simulink model "MinsegControlProjectSim"  (R2023a)
settings: Solver=FixedStepDiscrete  StartTime=0.0  StopTime=inf  FixedStep=0.03  RelTol=1e-3
values from neighbouring files (symbols this model uses):
  K_LQR = lqr(A,B,Q,R)    [MinsegControlProject.m]
libraries: arduinolib x2, RASPlib x2, simulink x1, MinSegLibrary_MinSegMega x1
settings Model: SimulationMode=external  ExtModeTrigDuration=2  Creator=nicho  LastModifiedBy=nicho
settings OptimizationCC: EnhancedBackFolding=on  PassReuseOutputArgsAs=Individual arguments  ZeroExternalMemoryAtStartup=off  ZeroInternalMemoryAtStartup=off  MaxStackSize=64  OptimizeBlockOrder=speed  DifferentSizesBufferReuse=on  OptimizationCustomize=off  EfficientTunableParamExpr=on
settings DebuggingCC: ParameterTunabilityLossMsg=error
settings HardwareCC: ProdBitPerInt=16  ProdBitPerPointer=16  ProdBitPerSizeT=16  ProdBitPerPtrDiffT=16  ProdLargestAtomicFloat=None  ProdWordSize=8  ProdHWDeviceType=Atmel->AVR  UseEmbeddedCoderFeatures=off  UseSimulinkCoderFeatures=off
settings SFSimCC: MATLABDynamicMemAlloc=off
settings RTWCC: Description=Embedded Coder  SystemTargetFile=ert.tlc  HardwareBoard=Arduino Mega 2560  TemplateMakefile=ert_default_tmf  RTWVerbose=off  Toolchain=Arduino AVR
settings CodeAppCC: ForceParamTrailComments=on  OperatorAnnotations=on  SimulinkDataObjDesc=on  SFDataObjDesc=on  MangleLength=10  InsertBlockDesc=on
settings ERTTargetCC: SupportContinuousTime=on  SupportNonInlinedSFcns=on  SupportVariableSizeSignals=on  ExtMode=on  ExtModeTransport=3  ExtModeStaticAlloc=on  ExtModeAutomaticAllocSize=off  ExtModeStaticAllocSize=2048  ExtModeMexFile=ext_xcp  ExtModeMexArgs=0 3 921600  ExtModeIntrfLevel=Level2 - Open  ERTSrcFileBannerTemplate=codertarget_code_template.cgt  ERTHdrFileBannerTemplate=codertarget_code_template.cgt  ERTDataSrcFileTemplate=codertarget_code_template.cgt  ERTDataHdrFileTemplate=codertarget_code_template.cgt

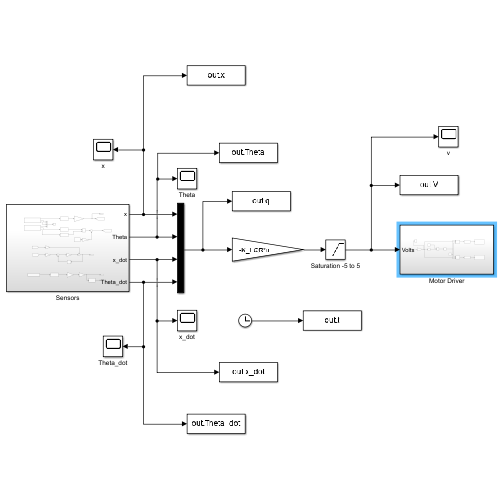
[thumbnail: Simulink's stored preview of the top-level diagram]
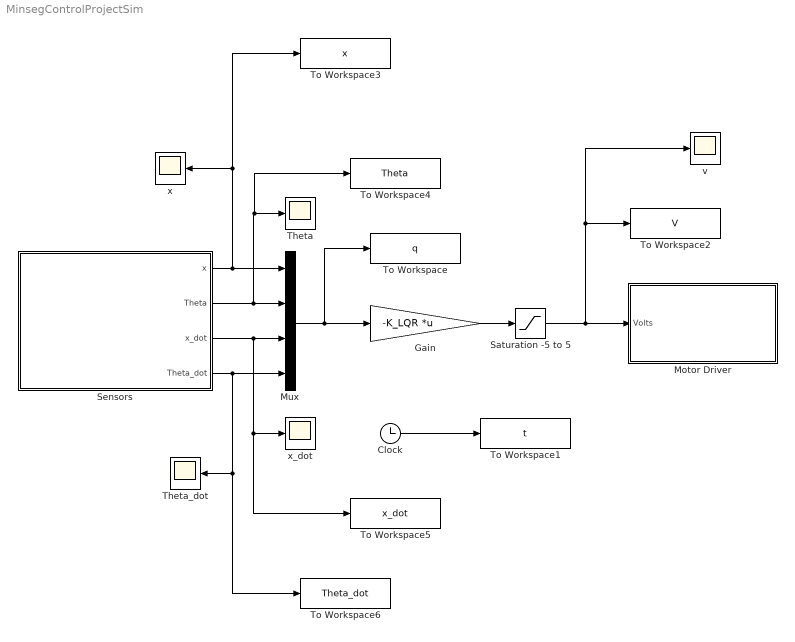
== system MinsegControlProjectSim ==
  Clock : Clock
  Gain : Gain  Gain=-K_LQR  Multiplication=Matrix(K*u)
  Motor Driver : Subsystem
  Mux : Mux
  Saturation -5 to 5 : Saturate  UpperLimit=5  LowerLimit=-5  LinearizeAsGain=off
  Sensors : Subsystem
  Theta : Scope
  Theta_dot : Scope
  To Workspace : ToWorkspace  VariableName=q  SampleTime=-1
      settings: Save2DSignal=2-D array (concatenate along first dimension)
  To Workspace1 : ToWorkspace  VariableName=t  SampleTime=-1
      settings: Save2DSignal=2-D array (concatenate along first dimension)
  To Workspace2 : ToWorkspace  VariableName=V  SampleTime=-1
      settings: Save2DSignal=2-D array (concatenate along first dimension)
  To Workspace3 : ToWorkspace  VariableName=x  SampleTime=-1
      settings: Save2DSignal=2-D array (concatenate along first dimension)
  To Workspace4 : ToWorkspace  VariableName=Theta  SampleTime=-1
      settings: Save2DSignal=2-D array (concatenate along first dimension)
  To Workspace5 : ToWorkspace  VariableName=x_dot  SampleTime=-1
      settings: Save2DSignal=2-D array (concatenate along first dimension)
  To Workspace6 : ToWorkspace  VariableName=Theta_dot  SampleTime=-1
      settings: Save2DSignal=2-D array (concatenate along first dimension)
  v : Scope
  x : Scope
  x_dot : Scope
  wires:
  Sensors/1(x) -> To Workspace3/1, x/1, Mux/1
  Sensors/2(Theta) -> To Workspace4/1, Theta/1, Mux/2
  Sensors/3(x_dot) -> To Workspace5/1, x_dot/1, Mux/3
  Sensors/4(Theta_dot) -> To Workspace6/1, Theta_dot/1, Mux/4
  Mux/1 -> To Workspace/1, Gain/1
  Clock/1 -> To Workspace1/1
  Gain/1 -> Saturation -5 to 5/1
  Saturation -5 to 5/1 -> v/1, To Workspace2/1, Motor Driver/1(Volts)

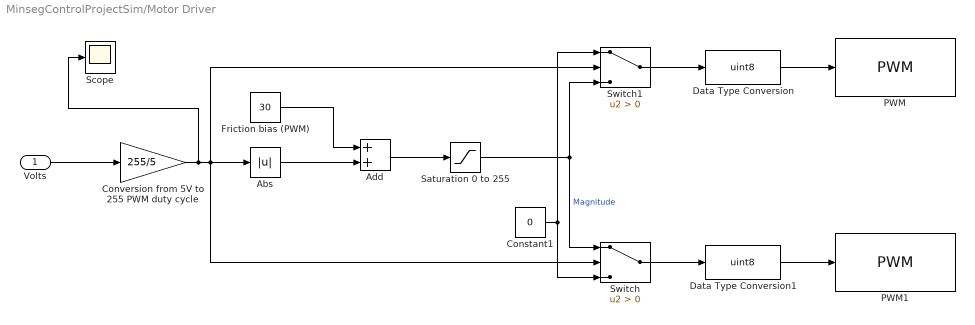
== system MinsegControlProjectSim/Motor Driver ==
  Volts : Inport
  Abs : Abs  SaturateOnIntegerOverflow=off
  Add : Sum
  Constant1 : Constant  Value=0
  Conversion from 5V to 255 PWM duty cycle : Gain  Gain=255/5
  Data Type Conversion : DataTypeConversion  OutDataTypeStr=uint8  SaturateOnIntegerOverflow=off  RndMeth=Floor
  Data Type Conversion1 : DataTypeConversion  OutDataTypeStr=uint8  SaturateOnIntegerOverflow=off  RndMeth=Floor
  Friction bias (PWM) : Constant  Value=30
  PWM : arduinolib/PWM  pinNumber=44  frequencyType=Default  desiredFrequency=490.2  achievableFrequency=490.2
  PWM1 : arduinolib/PWM  pinNumber=45  frequencyType=Default  desiredFrequency=490.2  achievableFrequency=490.2
  Saturation 0 to 255 : Saturate  UpperLimit=255  LowerLimit=0
  Scope : Scope
  Switch : Switch  Criteria=u2 > Threshold  SaturateOnIntegerOverflow=off  InputSameDT=off
  Switch1 : Switch  Criteria=u2 > Threshold  SaturateOnIntegerOverflow=off  InputSameDT=off
  wires:
  Friction bias (PWM)/1 -> Add/1
  Abs/1 -> Add/2
  Conversion from 5V to 255 PWM duty cycle/1 -> Scope/1, Switch/2, Switch1/2, Abs/1
  Volts/1 -> Conversion from 5V to 255 PWM duty cycle/1
  Constant1/1 -> Switch1/1, Switch/3
  Data Type Conversion1/1 -> PWM1/1
  Saturation 0 to 255/1 -> Switch1/3, Switch/1  "Magnitude"
  Add/1 -> Saturation 0 to 255/1
  Switch1/1 -> Data Type Conversion/1
  Data Type Conversion/1 -> PWM/1
  Switch/1 -> Data Type Conversion1/1

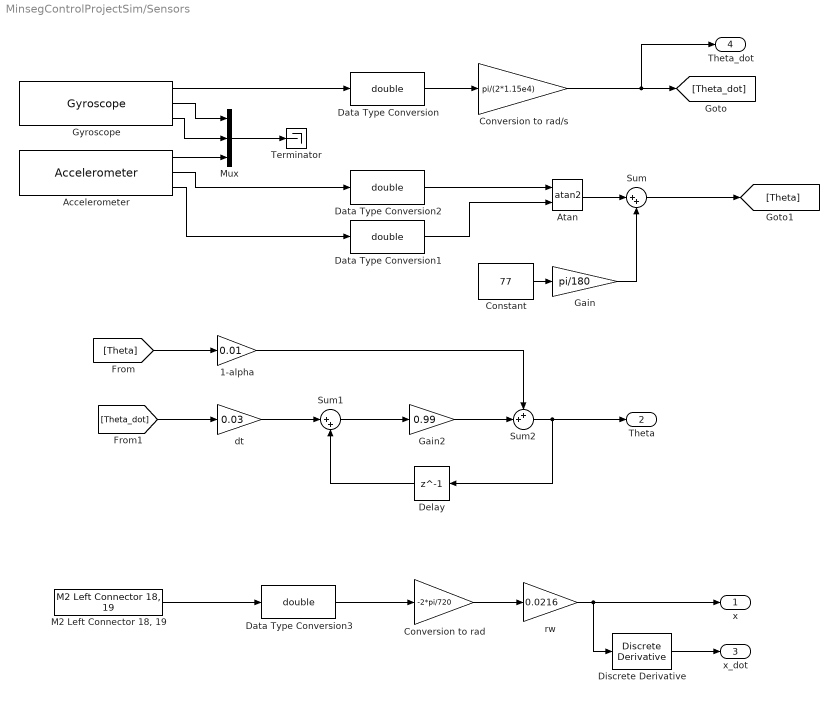
== system MinsegControlProjectSim/Sensors ==
  1-alpha : Gain  Gain=0.01
  Accelerometer : RASPlib/Accelerometer  SimulateUsing=Code generation
      settings: SourceProductName=Rensselaer Arduino Support Package
  Atan : Trigonometry  Operator=atan2
  Constant : Constant  Value=77
  Conversion to rad : Gain  Gain=-2*pi/720
  Conversion to rad/s : Gain  Gain=pi/(2*1.15e4)
  Data Type Conversion{,1..3} (4 alike) : DataTypeConversion  OutDataTypeStr=double  SaturateOnIntegerOverflow=off  RndMeth=Floor
  Delay : Delay  DelayLength=1
  Discrete Derivative : simulink/Discrete/Discrete Derivative  gainval=1.0  ICPrevScaledInput=0.0  OutMin=[]  OutMax=[]  OutDataType=fixdt(1, 16)  OutScaling=2^-10  DoSatur=off
  Gain : Gain  Gain=pi/180
  Gain2 : Gain  Gain=0.99
  Gyroscope : RASPlib/Gyroscope  DLPFmode=3
      settings: SourceProductName=Rensselaer Arduino Support Package
  "M2 Left Connector 18, 19" : MinSegLibrary_MinSegMega/M2 Left Connector 18, 19  Encoder=1  PinA=19  PinB=18
      settings: SourceProductName=Rensselaer Arduino Support Package
  Mux : Mux  Inputs=3
  Sum : Sum  Inputs=|++
  Sum1 : Sum  Inputs=|++
  Sum2 : Sum  Inputs=++|
  Terminator : Terminator
  dt : Gain  Gain=0.03
  rw : Gain  Gain=0.0216
  x : Outport
  Theta : Outport  Port=2
  x_dot : Outport  Port=3
  Theta_dot : Outport  Port=4
  wires:
  Sum2/1 -> Delay/1, Theta/1
  Mux/1 -> Terminator/1
  Gyroscope/3 -> Mux/2
  Gyroscope/2 -> Mux/1
  Accelerometer/1 -> Mux/3
  Discrete Derivative/1 -> x_dot/1
  Gyroscope/1 -> Data Type Conversion/1
  Data Type Conversion1/1 -> Atan/2
  Constant/1 -> Gain/1
  rw/1 -> x/1, Discrete Derivative/1
  Delay/1 -> Sum1/2
  Data Type Conversion2/1 -> Atan/1
  Accelerometer/2 -> Data Type Conversion2/1
  Atan/1 -> Sum/1
  Accelerometer/3 -> Data Type Conversion1/1
  Data Type Conversion/1 -> Conversion to rad/s/1
  [Theta_dot] -> dt/1
  [Theta] -> 1-alpha/1
  Sum1/1 -> Gain2/1
  Conversion to rad/1 -> rw/1
  dt/1 -> Sum1/1
  Gain2/1 -> Sum2/2
  "M2 Left Connector 18, 19"/1 -> Data Type Conversion3/1
  Data Type Conversion3/1 -> Conversion to rad/1
  Conversion to rad/s/1 -> Theta_dot/1, [Theta_dot]
  Sum/1 -> [Theta]
  Gain/1 -> Sum/2
  1-alpha/1 -> Sum2/1
